simulink model "power_circ2ss_slk"  (Simulink 6.0)
settings: Solver=ode15s  SolverMode=SingleTasking  StartTime=0.0  StopTime=0.25  RelTol=1e-4  AbsTol=1e-6
InitFcn:
  | power_circ2ss
undefined symbols (not defined in the file or in its folder): A, B, C, D, x0
libraries: powerlib_models x2, powerlib_extras x1
settings Model: Creator=patrice  LastModifiedBy=batserve  ExtModeTrigMode=oneshot  ExtModeArmWhenConnect=off  ExtModeAutoUpdateStatusClock=off
settings DataIOCC: LimitDataPoints=off  SignalLoggingName=sigsOut
settings OptimizationCC: BlockReduction=off  BooleanDataType=off
settings DebuggingCC: SolverPrmCheckMsg=none
settings HardwareCC: TargetUnknown=on

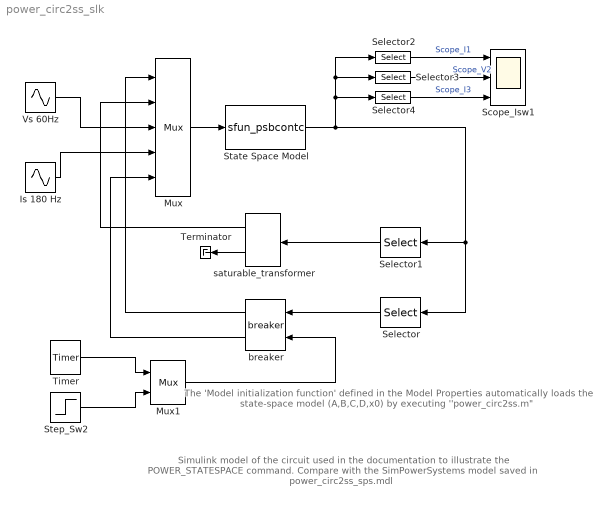
== system power_circ2ss_slk ==
  note: The 'Model  initialization function' defined in the
      | Model Properties automatically
      | loads the state-space model (A,B,C,D,x0)
      | by executing  ''power_circ2ss.m"
  note: Simulink model of the circuit used in the documentation to illustrate the POWER_STATESPACE command.
      | Compare with the SimPowerSystems model saved in power_circ2ss_sps.mdl
  Is 180 Hz : Sin  Amplitude=2  Frequency=2*pi*180  Phase=-30*pi/180  SampleTime=0
  Mux : Mux  Inputs=[2 1 1 1 2]
  Mux1 : Mux  Inputs=2
  Scope_Isw1 : Scope  NumInputPorts=3
      settings: TickLabels=on  TimeRange=0.25  YMin=-15~-400~-400  YMax=10~200~200  DataFormat=Array
  Selector : Selector  Orientation=left  Elements=[1 2]  InputPortWidth=8
  Selector1 : Selector  Orientation=left  Elements=5  InputPortWidth=8
  Selector2 : Selector  Elements=6  InputPortWidth=8
  Selector3 : Selector  Elements=7  InputPortWidth=8
  Selector4 : Selector  Elements=8  InputPortWidth=8
  State Space Model : S-Function  FunctionName=sfun_psbcontc  Parameters=A,B,C,D,x0, [0.01; 0.1], [0 0]
  Step_Sw2 : Step  Time=0.05  SampleTime=0
  Terminator : Terminator
  Timer : powerlib_extras/Control  Blocks/Timer  t=[0 100e-3 130e-3]  e=[1 0 1 ]
  Vs 60Hz : Sin  Amplitude=100  Frequency=2*pi*60  SampleTime=0
  breaker : powerlib_models/Continuous/breaker  Orientation=left  Nsw=2  istate=[1 0]  Rsw=[0.01 0.1]
  saturable_transformer : powerlib_models/Continuous/saturable_transformer  Orientation=left  SaturationFlux=[-0.4877 -0.4502 0.4502 0.4877]  SaturationCurrent=[-141.4 -0.1414 0.1414 141.4]  InitialFlux=-0.2707
  wires:
  Mux/1 -> State Space Model/1
  Step_Sw2/1 -> Mux1/2
  Mux1/1 -> breaker/2
  Timer/1 -> Mux1/1
  breaker/1 -> Mux/1
  saturable_transformer/1 -> Mux/2
  Vs 60Hz/1 -> Mux/3
  Is 180 Hz/1 -> Mux/4
  breaker/2 -> Mux/5
  Selector/1 -> breaker/1
  Selector1/1 -> saturable_transformer/1
  State Space Model/1 -> Selector/1, Selector1/1, Selector2/1, Selector3/1, Selector4/1
  Selector2/1 -> Scope_Isw1/1  "Scope_I1"
  Selector3/1 -> Scope_Isw1/2  "Scope_V2"
  Selector4/1 -> Scope_Isw1/3  "Scope_I3"
  saturable_transformer/2 -> Terminator/1
